simulink model "week3_1"  (R2020b)
settings: Solver=VariableStepAuto  StartTime=0.0  StopTime=10.0  RelTol=1e-3
settings Model: Creator=lalit  LastModifiedBy=lalit

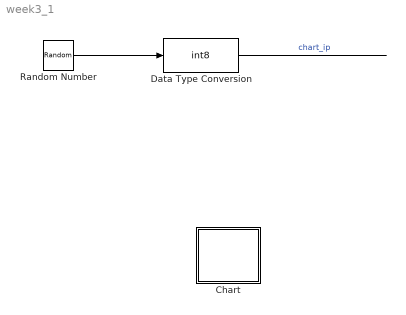
== system week3_1 ==
  Chart : Stateflow chart  TreatAsAtomicUnit=on
  Data Type Conversion : DataTypeConversion  OutDataTypeStr=int8  RndMeth=Nearest  SaturateOnIntegerOverflow=on
  Random Number : RandomNumber  SampleTime=0.1
  wires:
  Random Number/1 -> Data Type Conversion/1
  Data Type Conversion/1 -> ?  "chart_ip"

== stateflow chart week3_1/Chart ==
  state coins_inserted
  state no_coins
  (default) -> no_coins
